simulink model "Final_Conveyor"  (Simulink 8.3)
settings: Solver=ode45  StartTime=0.0  StopTime=9000.0  RelTol=1e-3
undefined symbols (not defined in the file or in its folder): rc_input, rc_LLC, rc_LLC1, rc_LLC2, rc_LLC3, rc_LLC4, rc_LLC5, rc_output, rc_switch_2TO1, rc_swith_1TO1, rc_sysAct, rc_sysAct1, rc_sysAct2, rc_sysAct3, rc_sysAct4, rc_sysAct5
settings Model: Creator=obo  LastModifiedBy=obo
settings DataIOCC: SignalLoggingSaveFormat=Dataset
settings DebuggingCC: UnderspecifiedInitializationDetection=Simplified  StateNameClashWarn=none
settings GRTTargetCC: CombineOutputUpdateFcns=on  GRTInterface=off

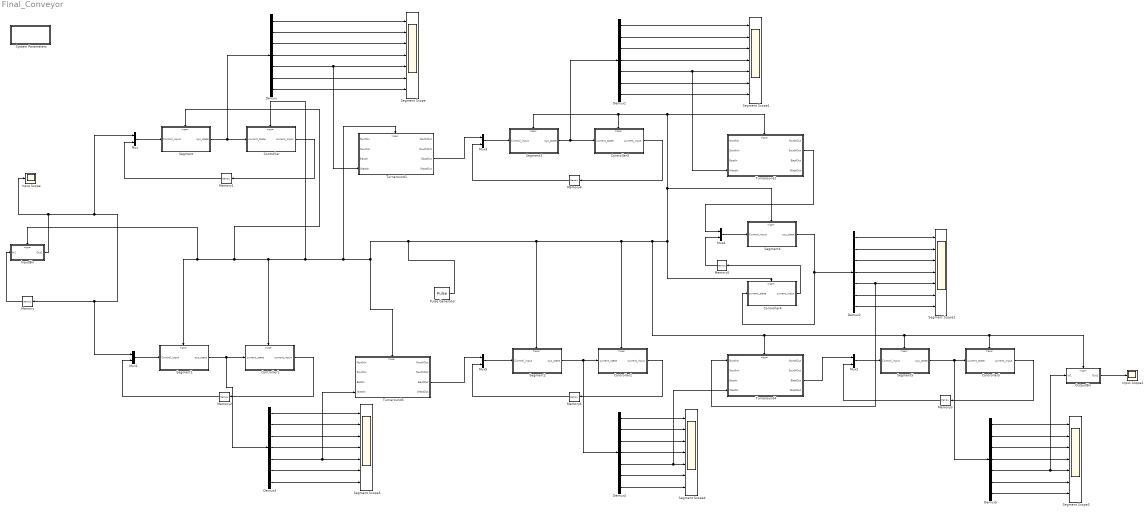
== system Final_Conveyor ==
  Controller : Subsystem  TreatAsAtomicUnit=on
  Controller1 : Subsystem  TreatAsAtomicUnit=on
  Controller2 : Subsystem  TreatAsAtomicUnit=on
  Controller3 : Subsystem  TreatAsAtomicUnit=on
  Controller4 : Subsystem  TreatAsAtomicUnit=on
  Controller5 : Subsystem  TreatAsAtomicUnit=on
  Demux{,1..5} (6 alike) : Demux  Outputs=7
  Input Scope : Scope
      settings: YMin=75  YMax=600
  Input Scope2 : Scope
      settings: TimeRange=9000  YMin=-250  YMax=450  SaveName=ScopeData5
  InputBin : Subsystem
  Memory{,1..6} (7 alike) : Memory
  Mux{,1..5} (6 alike) : Mux  Inputs=2
  OutputBin : Subsystem
  Pulse Generator : DiscretePulseGenerator  PulseType=Time based  Period=1  PulseWidth=50  PhaseDelay=0.01
  Segment : Subsystem  TreatAsAtomicUnit=on
  Segment Scope{,1..5} (6 alike) : Scope  NumInputPorts=7
      Segment Scope settings: TimeRange=9000  YMin=100~100~200~2.77556e-17~100~0.2~-20  YMax=550~550~1000~0.5~550~1~20  MaxDataPoints=10000
      Segment Scope1 settings: TimeRange=9000  YMin=100~100~200~2.77556e-17~100~0.2~-40  YMax=700~700~1000~0.5~700~1~60  SaveName=ScopeData2  MaxDataPoints=10000
      Segment Scope2 settings: TimeRange=9000  YMin=100~100~200~2.77556e-17~100~0.2~-75  YMax=700~700~1000~0.5~700~1~75  SaveName=ScopeData3  MaxDataPoints=10000
      Segment Scope3 settings: TimeRange=9000  YMin=300~300~500~0.05~300~0.3~-100  YMax=1100~1100~2000~0.5~1100~1~100  SaveName=ScopeData4  MaxDataPoints=10000
      Segment Scope4 settings: TimeRange=9000  YMin=0~0~2~5~5.55112e-17~0~0.2  YMax=35~150~8~25~1~700~1  SaveName=ScopeData6  MaxDataPoints=10000
      Segment Scope5 settings: TimeRange=9000  YMin=200~200~400~0.05~200~0.4~-40  YMax=650~650~1000~0.5~650~1~30  SaveName=ScopeData7  MaxDataPoints=10000
  Segment1 : Subsystem  TreatAsAtomicUnit=on
  Segment2 : Subsystem  TreatAsAtomicUnit=on
  Segment3 : Subsystem  TreatAsAtomicUnit=on
  Segment4 : Subsystem  TreatAsAtomicUnit=on
  Segment5 : Subsystem  TreatAsAtomicUnit=on
  System Parameters : Subsystem  mask(Initialization Block){}
      mask help: Calls sc_init.m on it's initialization to declare and initialize all global variables.
      mask init:
      | rc_init
      mask Display: disp('Initialization')
  "Turnaround1 " : Subsystem
  Turnaround2 : Subsystem
  Turnaround3 : Subsystem
  "Turnaround4 " : Subsystem
  wires:
  InputBin/1(Out1) -> Mux/1, Mux1/1, Memory/1, Input Scope/1
  Memory/1 -> InputBin/1(In1)
  Segment/1(sys_state) -> Demux/1, Controller/1(current_state)
  Controller/1(current_input) -> Memory1/1
  Memory1/1 -> Mux/2
  Mux/1 -> Segment/1(Control_input)
  Segment1/1(sys_state) -> Demux3/1, Controller1/1(current_state)
  Controller1/1(current_input) -> Memory2/1
  Memory2/1 -> Mux1/2
  Mux1/1 -> Segment1/1(Control_input)
  "Turnaround4 "/3(EastOut) -> Mux2/1
  Segment5/1(sys_state) -> Demux5/1, Controller5/1(current_state)
  Controller5/1(current_input) -> Memory3/1
  Memory3/1 -> Mux2/2
  Mux2/1 -> Segment5/1(Control_input)
  OutputBin/1(Out1) -> Input Scope2/1
  Segment3/1(sys_state) -> Demux1/1, Controller3/1(current_state)
  Controller3/1(current_input) -> Memory4/1
  Memory4/1 -> Mux3/2
  Mux3/1 -> Segment3/1(Control_input)
  "Turnaround1 "/3(EastOut) -> Mux3/1
  Segment4/1(sys_state) -> Demux2/1, Controller4/1(current_state)
  Controller4/1(current_input) -> Memory5/1
  Memory5/1 -> Mux4/2
  Mux4/1 -> Segment4/1(Control_input)
  Turnaround2/2(SouthOut) -> Mux4/1
  Segment2/1(sys_state) -> Demux4/1, Controller2/1(current_state)
  Controller2/1(current_input) -> Memory6/1
  Memory6/1 -> Mux5/2
  Mux5/1 -> Segment2/1(Control_input)
  Turnaround3/3(EastOut) -> Mux5/1
  Pulse Generator/1 -> Turnaround3/Trigger, Segment1/Trigger, InputBin/Trigger, Segment/Trigger, Controller1/Trigger, Controller/Trigger, "Turnaround1 "/Trigger, Controller3/Trigger, Segment3/Trigger, Turnaround2/Trigger, Segment4/Trigger, Controller4/Trigger, "Turnaround4 "/Trigger, OutputBin/Trigger, Controller5/Trigger, Segment5/Trigger, Controller2/Trigger, Segment2/Trigger
  Demux/7 -> Segment Scope/7
  Demux/1 -> Segment Scope/1
  Demux/2 -> Segment Scope/2
  Demux/3 -> Segment Scope/3
  Demux/4 -> Segment Scope/4
  Demux/5 -> "Turnaround1 "/4(WestIn), Segment Scope/5
  Demux/6 -> Segment Scope/6
  Demux1/3 -> Segment Scope1/3
  Demux1/1 -> Segment Scope1/1
  Demux1/2 -> Segment Scope1/2
  Demux1/4 -> Segment Scope1/4
  Demux1/5 -> Turnaround2/4(WestIn), Segment Scope1/5
  Demux1/6 -> Segment Scope1/6
  Demux1/7 -> Segment Scope1/7
  Demux3/1 -> Segment Scope5/1
  Demux3/2 -> Segment Scope5/2
  Demux3/3 -> Segment Scope5/3
  Demux3/4 -> Segment Scope5/4
  Demux3/5 -> Turnaround3/4(WestIn), Segment Scope5/5
  Demux3/6 -> Segment Scope5/6
  Demux3/7 -> Segment Scope5/7
  Demux4/1 -> Segment Scope4/1
  Demux4/2 -> Segment Scope4/2
  Demux4/3 -> Segment Scope4/3
  Demux4/4 -> Segment Scope4/4
  Demux4/5 -> "Turnaround4 "/4(WestIn), Segment Scope4/5
  Demux4/6 -> Segment Scope4/6
  Demux4/7 -> Segment Scope4/7
  Demux2/1 -> Segment Scope2/1
  Demux2/2 -> Segment Scope2/2
  Demux2/3 -> Segment Scope2/3
  Demux2/4 -> Segment Scope2/4
  Demux2/5 -> "Turnaround4 "/1(NorthIn), Segment Scope2/5
  Demux2/6 -> Segment Scope2/6
  Demux2/7 -> Segment Scope2/7
  Demux5/1 -> Segment Scope3/1
  Demux5/2 -> Segment Scope3/2
  Demux5/3 -> Segment Scope3/3
  Demux5/4 -> Segment Scope3/4
  Demux5/5 -> OutputBin/1(In1), Segment Scope3/5
  Demux5/6 -> Segment Scope3/6
  Demux5/7 -> Segment Scope3/7

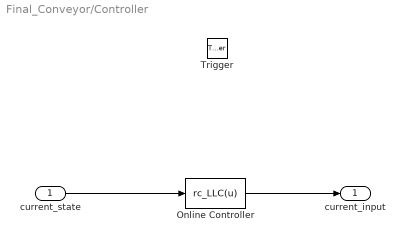
== system Final_Conveyor/Controller ==
  current_state : Inport
  Trigger : TriggerPort  TriggerType=falling  PortDimensions=1
  Online Controller : MATLABFcn  MATLABFcn=rc_LLC(u)  OutputDimensions=1  Output1D=off
  current_input : Outport  InitialOutput=0
  wires:
  Online Controller/1 -> current_input/1
  current_state/1 -> Online Controller/1

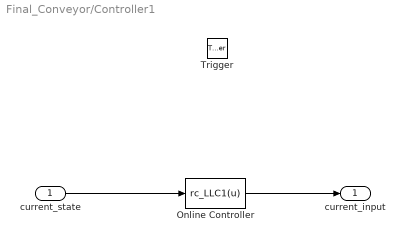
== system Final_Conveyor/Controller1 ==
  current_state : Inport
  Trigger : TriggerPort  TriggerType=falling  PortDimensions=1
  Online Controller : MATLABFcn  MATLABFcn=rc_LLC1(u)  OutputDimensions=1  Output1D=off
  current_input : Outport  InitialOutput=0
  wires:
  Online Controller/1 -> current_input/1
  current_state/1 -> Online Controller/1

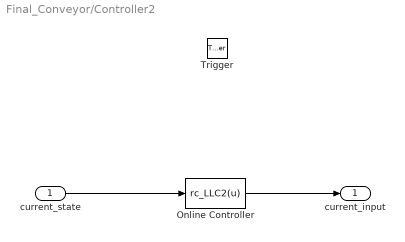
== system Final_Conveyor/Controller2 ==
  current_state : Inport
  Trigger : TriggerPort  TriggerType=falling  PortDimensions=1
  Online Controller : MATLABFcn  MATLABFcn=rc_LLC2(u)  OutputDimensions=1  Output1D=off
  current_input : Outport  InitialOutput=0
  wires:
  Online Controller/1 -> current_input/1
  current_state/1 -> Online Controller/1

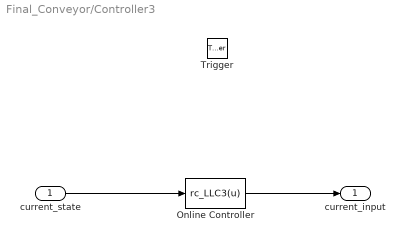
== system Final_Conveyor/Controller3 ==
  current_state : Inport
  Trigger : TriggerPort  TriggerType=falling  PortDimensions=1
  Online Controller : MATLABFcn  MATLABFcn=rc_LLC3(u)  OutputDimensions=1  Output1D=off
  current_input : Outport  InitialOutput=0
  wires:
  Online Controller/1 -> current_input/1
  current_state/1 -> Online Controller/1

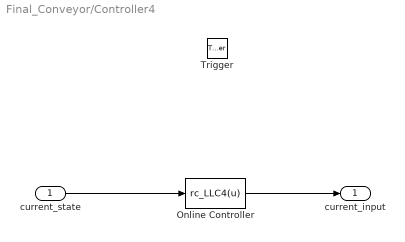
== system Final_Conveyor/Controller4 ==
  current_state : Inport
  Trigger : TriggerPort  TriggerType=falling  PortDimensions=1
  Online Controller : MATLABFcn  MATLABFcn=rc_LLC4(u)  OutputDimensions=1  Output1D=off
  current_input : Outport  InitialOutput=0
  wires:
  Online Controller/1 -> current_input/1
  current_state/1 -> Online Controller/1

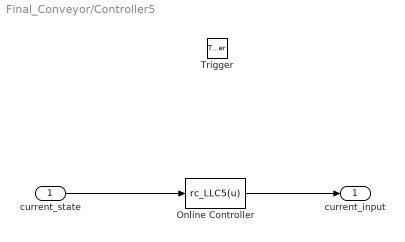
== system Final_Conveyor/Controller5 ==
  current_state : Inport
  Trigger : TriggerPort  TriggerType=falling  PortDimensions=1
  Online Controller : MATLABFcn  MATLABFcn=rc_LLC5(u)  OutputDimensions=1  Output1D=off
  current_input : Outport  InitialOutput=0
  wires:
  Online Controller/1 -> current_input/1
  current_state/1 -> Online Controller/1

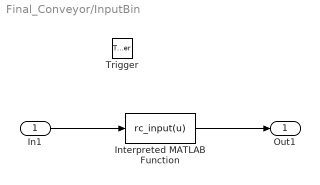
== system Final_Conveyor/InputBin ==
  In1 : Inport
  Trigger : TriggerPort  TriggerType=falling  PortDimensions=1
  Interpreted MATLAB Function : MATLABFcn  MATLABFcn=rc_input(u)  OutputDimensions=1
  Out1 : Outport  InitialOutput=[0]
  wires:
  In1/1 -> Interpreted MATLAB Function/1
  Interpreted MATLAB Function/1 -> Out1/1

== system Final_Conveyor/OutputBin ==
  In1 : Inport
  Trigger : TriggerPort  TriggerType=falling  PortDimensions=1
  Interpreted MATLAB Function : MATLABFcn  MATLABFcn=rc_output(u)
  Out1 : Outport  InitialOutput=[0]
  wires:
  In1/1 -> Interpreted MATLAB Function/1
  Interpreted MATLAB Function/1 -> Out1/1

== system Final_Conveyor/Segment ==
  Control_input : Inport
  Trigger : TriggerPort  PortDimensions=1
  Physical system : MATLABFcn  MATLABFcn=rc_sysAct(u)  OutputDimensions=1*7  Output1D=off
  sys_state : Outport  InitialOutput=0
  wires:
  Control_input/1 -> Physical system/1
  Physical system/1 -> sys_state/1

== system Final_Conveyor/Segment1 ==
  Control_input : Inport
  Trigger : TriggerPort  PortDimensions=1
  Physical system : MATLABFcn  MATLABFcn=rc_sysAct1(u)  OutputDimensions=1*7  Output1D=off
  sys_state : Outport  InitialOutput=0
  wires:
  Control_input/1 -> Physical system/1
  Physical system/1 -> sys_state/1

== system Final_Conveyor/Segment2 ==
  Control_input : Inport
  Trigger : TriggerPort  PortDimensions=1
  Physical system : MATLABFcn  MATLABFcn=rc_sysAct2(u)  OutputDimensions=1*7  Output1D=off
  sys_state : Outport  InitialOutput=0
  wires:
  Control_input/1 -> Physical system/1
  Physical system/1 -> sys_state/1

== system Final_Conveyor/Segment3 ==
  Control_input : Inport
  Trigger : TriggerPort  PortDimensions=1
  Physical system : MATLABFcn  MATLABFcn=rc_sysAct3(u)  OutputDimensions=1*7  Output1D=off
  sys_state : Outport  InitialOutput=0
  wires:
  Control_input/1 -> Physical system/1
  Physical system/1 -> sys_state/1

== system Final_Conveyor/Segment4 ==
  Control_input : Inport
  Trigger : TriggerPort  PortDimensions=1
  Physical system : MATLABFcn  MATLABFcn=rc_sysAct4(u)  OutputDimensions=1*7  Output1D=off
  sys_state : Outport  InitialOutput=0
  wires:
  Control_input/1 -> Physical system/1
  Physical system/1 -> sys_state/1

== system Final_Conveyor/Segment5 ==
  Control_input : Inport
  Trigger : TriggerPort  PortDimensions=1
  Physical system : MATLABFcn  MATLABFcn=rc_sysAct5(u)  OutputDimensions=1*7  Output1D=off
  sys_state : Outport  InitialOutput=0
  wires:
  Control_input/1 -> Physical system/1
  Physical system/1 -> sys_state/1

== system Final_Conveyor/System Parameters ==

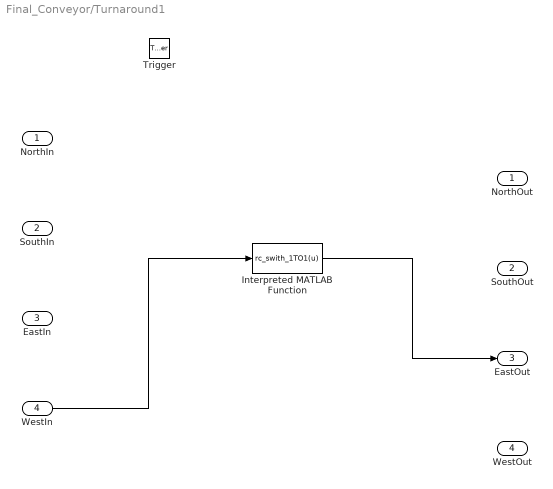
== system Final_Conveyor/Turnaround1  ==
  NorthIn : Inport
  SouthIn : Inport  Port=2
  EastIn : Inport  Port=3
  WestIn : Inport  Port=4
  Trigger : TriggerPort  TriggerType=falling  PortDimensions=1
  Interpreted MATLAB Function : MATLABFcn  MATLABFcn=rc_swith_1TO1(u)
  NorthOut : Outport  InitialOutput=[0]
  SouthOut : Outport  Port=2  InitialOutput=[0]
  EastOut : Outport  Port=3  InitialOutput=[0]
  WestOut : Outport  Port=4  InitialOutput=[0]
  wires:
  WestIn/1 -> Interpreted MATLAB Function/1
  Interpreted MATLAB Function/1 -> EastOut/1

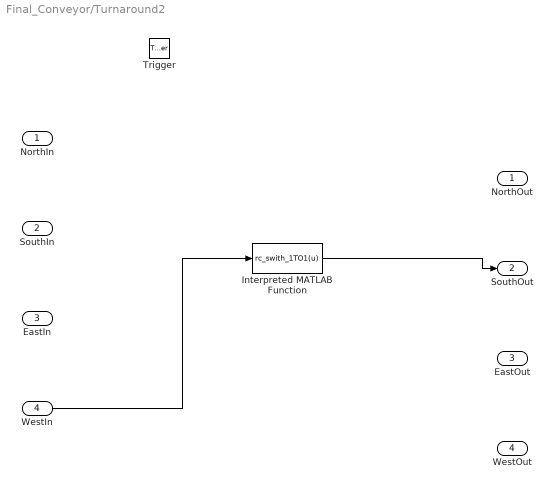
== system Final_Conveyor/Turnaround2 ==
  NorthIn : Inport
  SouthIn : Inport  Port=2
  EastIn : Inport  Port=3
  WestIn : Inport  Port=4
  Trigger : TriggerPort  TriggerType=falling  PortDimensions=1
  Interpreted MATLAB Function : MATLABFcn  MATLABFcn=rc_swith_1TO1(u)
  NorthOut : Outport  InitialOutput=[0]
  SouthOut : Outport  Port=2  InitialOutput=[0]
  EastOut : Outport  Port=3  InitialOutput=[0]
  WestOut : Outport  Port=4  InitialOutput=[0]
  wires:
  WestIn/1 -> Interpreted MATLAB Function/1
  Interpreted MATLAB Function/1 -> SouthOut/1

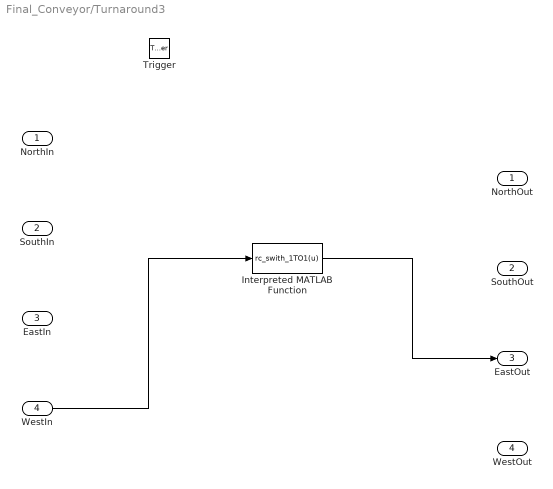
== system Final_Conveyor/Turnaround3 ==
  NorthIn : Inport
  SouthIn : Inport  Port=2
  EastIn : Inport  Port=3
  WestIn : Inport  Port=4
  Trigger : TriggerPort  TriggerType=falling  PortDimensions=1
  Interpreted MATLAB Function : MATLABFcn  MATLABFcn=rc_swith_1TO1(u)
  NorthOut : Outport  InitialOutput=[0]
  SouthOut : Outport  Port=2  InitialOutput=[0]
  EastOut : Outport  Port=3  InitialOutput=[0]
  WestOut : Outport  Port=4  InitialOutput=[0]
  wires:
  WestIn/1 -> Interpreted MATLAB Function/1
  Interpreted MATLAB Function/1 -> EastOut/1

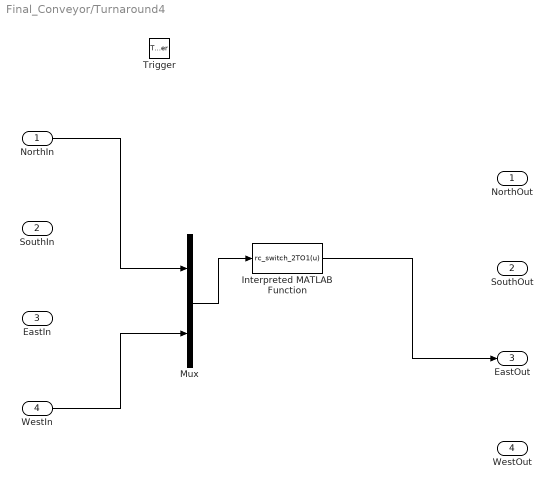
== system Final_Conveyor/Turnaround4  ==
  NorthIn : Inport
  SouthIn : Inport  Port=2
  EastIn : Inport  Port=3
  WestIn : Inport  Port=4
  Trigger : TriggerPort  TriggerType=falling  PortDimensions=1
  Interpreted MATLAB Function : MATLABFcn  MATLABFcn=rc_switch_2TO1(u)
  Mux : Mux  Inputs=2
  NorthOut : Outport  InitialOutput=[0]
  SouthOut : Outport  Port=2  InitialOutput=[0]
  EastOut : Outport  Port=3  InitialOutput=[0]
  WestOut : Outport  Port=4  InitialOutput=[0]
  wires:
  WestIn/1 -> Mux/2
  NorthIn/1 -> Mux/1
  Mux/1 -> Interpreted MATLAB Function/1
  Interpreted MATLAB Function/1 -> EastOut/1
